simulink model "sldemo_variant_subsystems_enum"  (Simulink 7.6)
settings: Solver=FixedStepDiscrete  StartTime=0.0  StopTime=10.0  RelTol=1e-3
PreLoadFcn:
  | VSSE_NONLINEAR_CONTROLLER=Simulink.Variant('VSSE_MODE==sldemo_vss_CONTROLLER_TYPE.NONLINEAR')
  | VSSE_SECOND_ORDER_CONTROLLER=Simulink.Variant('VSSE_MODE==sldemo_vss_CONTROLLER_TYPE.SECOND_ORDER')
  | 
  | VSSE_MODE=sldemo_vss_CONTROLLER_TYPE.SECOND_ORDER
  | 
  | VSSE_PROTOTYPE = Simulink.Variant('VSSE_CURRENT_BUILD==sldemo_vss_BUILD_TYPE.PROTOTYPE')
  | VSSE_PRODUCTION = Simulink.Variant('VSSE_CURRENT_BUILD==sldemo_vss_BUILD_TYPE.PRODUCTION')
  | 
  | VSSE_CURRENT_BUILD=sldemo_vss_BUILD_TYPE.PRODUCTION
Description:
  | Variant Subsystems - Enumerations and Reuse
  | 
  | This demo illustrates Simulink(R) variant subsystems using enumerations
  | with Simulink.Variant objects. Variant subsystems let you provide multiple
  | implementations to a subsystem where only one implementation is active
  | during simulation. You can programmatically swap out the active
  | implementation and replace it with one of the other implementations
  | without modifying the model.
settings Model: Creator=The MathWorks Inc.
settings DataIOCC: SaveFormat=StructureWithTime
settings OptimizationCC: InlineParams=on
settings RTWCC: ProcessScript=grt_make_rtw_hook
settings CodeAppCC: MaxIdLength=100

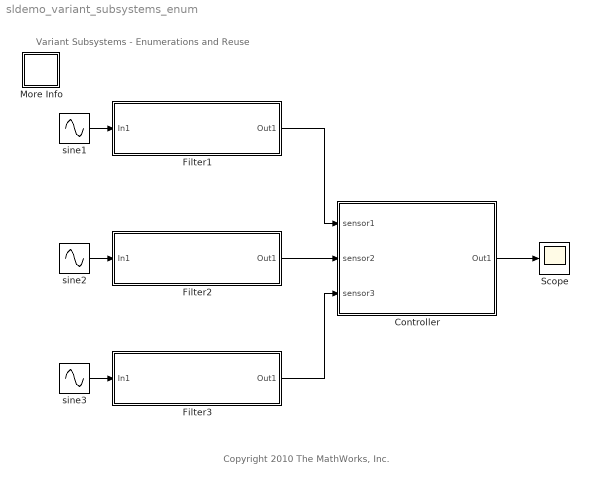
== system sldemo_variant_subsystems_enum ==
  note: Copyright 2010 The MathWorks, Inc.
  note: Variant Subsystems - Enumerations and Reuse
  Controller : Subsystem  Variant=on
  Filter1 : Subsystem  Variant=on
  Filter2 : Subsystem  Variant=on
  Filter3 : Subsystem  Variant=on
  More Info : Subsystem
      settings: OpenFcn=showdemo('sldemo_mdlref_variants')
      mask Display: disp('?')
  Scope : Scope
  sine1 : Sin  Amplitude=.1  Frequency=pi/3  SampleTime=.01
  sine2 : Sin  Amplitude=2  SampleTime=.01
  sine3 : Sin  Amplitude=.3  Frequency=pi/6  SampleTime=.01
  wires:
  sine2/1 -> Filter2/1(In1)
  sine1/1 -> Filter1/1(In1)
  sine3/1 -> Filter3/1(In1)
  Controller/1(Out1) -> Scope/1
  Filter3/1(Out1) -> Controller/3(sensor3)
  Filter2/1(Out1) -> Controller/2(sensor2)
  Filter1/1(Out1) -> Controller/1(sensor1)

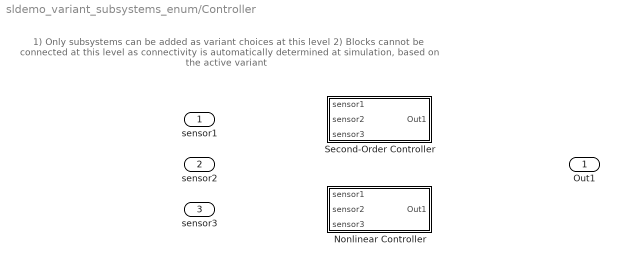
== system sldemo_variant_subsystems_enum/Controller ==
  note: 1) Only subsystems can be added as variant choices at this level
      | 2) Blocks cannot be connected at this level as connectivity is
      | automatically determined at simulation, based on the active variant
  sensor1 : Inport
  sensor2 : Inport  Port=2
  sensor3 : Inport  Port=3
  Nonlinear Controller : Subsystem  VariantObject=VSSE_NONLINEAR_CONTROLLER
  Second-Order Controller : Subsystem  VariantObject=VSSE_SECOND_ORDER_CONTROLLER
  Out1 : Outport

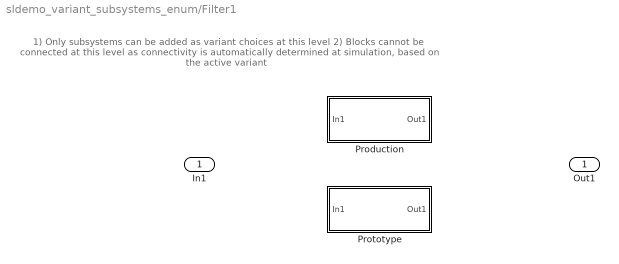
== system sldemo_variant_subsystems_enum/Filter1 ==
  note: 1) Only subsystems can be added as variant choices at this level
      | 2) Blocks cannot be connected at this level as connectivity is
      | automatically determined at simulation, based on the active variant
  In1 : Inport
  Production : Subsystem  VariantObject=VSSE_PRODUCTION
  Prototype : Subsystem  VariantObject=VSSE_PROTOTYPE
  Out1 : Outport

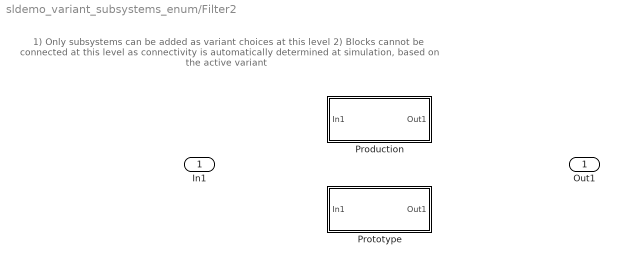
== system sldemo_variant_subsystems_enum/Filter2 ==
  note: 1) Only subsystems can be added as variant choices at this level
      | 2) Blocks cannot be connected at this level as connectivity is
      | automatically determined at simulation, based on the active variant
  In1 : Inport
  Production : Subsystem  VariantObject=VSSE_PRODUCTION
  Prototype : Subsystem  VariantObject=VSSE_PROTOTYPE
  Out1 : Outport

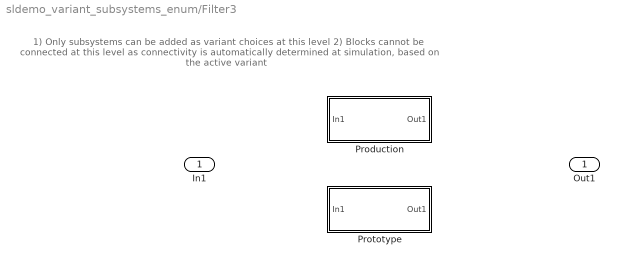
== system sldemo_variant_subsystems_enum/Filter3 ==
  note: 1) Only subsystems can be added as variant choices at this level
      | 2) Blocks cannot be connected at this level as connectivity is
      | automatically determined at simulation, based on the active variant
  In1 : Inport
  Production : Subsystem  VariantObject=VSSE_PRODUCTION
  Prototype : Subsystem  VariantObject=VSSE_PROTOTYPE
  Out1 : Outport

== system sldemo_variant_subsystems_enum/More Info ==
  note: Model Reference Variants - Enumerations and Reuse
  note: The following demo illustrates some Simulink.Variant capabilities
      |
      |    1. Enumerations: MATLAB enumeration classes can be used to improve
      |       readability in the conditions of the variant object.
      |
      |    2. Reuse: Simulink.Variant's can be reused in different Model blocks.

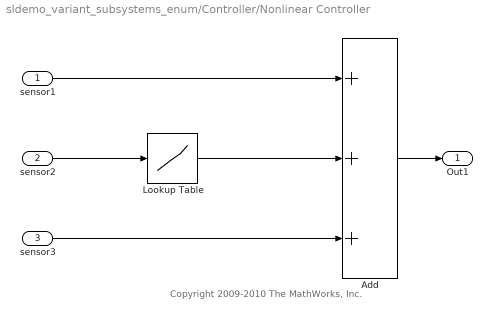
== system sldemo_variant_subsystems_enum/Controller/Nonlinear Controller ==
  note: Copyright 2009-2010 The MathWorks, Inc.
  sensor1 : Inport
  sensor2 : Inport  Port=2
  sensor3 : Inport  Port=3
  Add : Sum  Inputs=+++  SampleTime=.01
  Lookup Table : Lookup  InputValues=[-5:5]  Table=tanh([-5:5])
  Out1 : Outport
  wires:
  Add/1 -> Out1/1
  sensor1/1 -> Add/1
  sensor3/1 -> Add/3
  Lookup Table/1 -> Add/2
  sensor2/1 -> Lookup Table/1

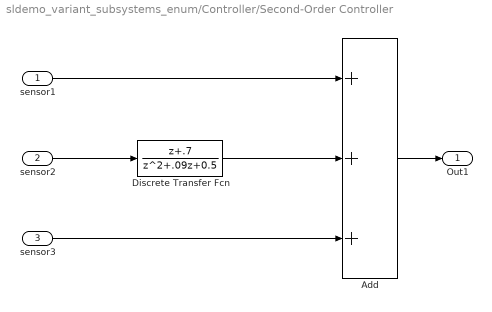
== system sldemo_variant_subsystems_enum/Controller/Second-Order Controller ==
  sensor1 : Inport
  sensor2 : Inport  Port=2
  sensor3 : Inport  Port=3
  Add : Sum  Inputs=+++
  Discrete Transfer Fcn : DiscreteTransferFcn  Numerator=[1 .7]  Denominator=[1 .09 0.5]  SampleTime=.01
  Out1 : Outport
  wires:
  Add/1 -> Out1/1
  sensor1/1 -> Add/1
  sensor3/1 -> Add/3
  Discrete Transfer Fcn/1 -> Add/2
  sensor2/1 -> Discrete Transfer Fcn/1

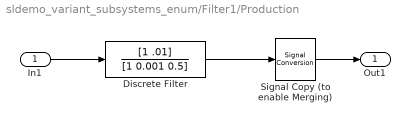
== system sldemo_variant_subsystems_enum/Filter1/Production ==
  In1 : Inport
  Discrete Filter : DiscreteFilter  Numerator=[1 .01]  Denominator=[1 0.001 0.5]  SampleTime=.01
  Signal Copy (to enable Merging) : SignalConversion  ConversionOutput=Contiguous copy
  Out1 : Outport
  wires:
  In1/1 -> Discrete Filter/1
  Discrete Filter/1 -> Signal Copy (to enable Merging)/1
  Signal Copy (to enable Merging)/1 -> Out1/1

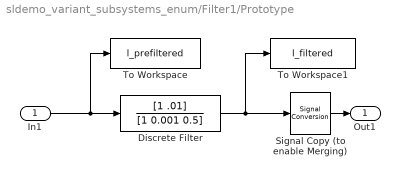
== system sldemo_variant_subsystems_enum/Filter1/Prototype ==
  In1 : Inport
  Discrete Filter : DiscreteFilter  Numerator=[1 .01]  Denominator=[1 0.001 0.5]  SampleTime=.01
  Signal Copy (to enable Merging) : SignalConversion  ConversionOutput=Contiguous copy
  To Workspace : ToWorkspace  VariableName=l_prefiltered  SampleTime=-1  SaveFormat=Structure
  To Workspace1 : ToWorkspace  VariableName=l_filtered  SampleTime=-1  SaveFormat=Structure
  Out1 : Outport
  wires:
  In1/1 -> To Workspace/1, Discrete Filter/1
  Discrete Filter/1 -> Signal Copy (to enable Merging)/1, To Workspace1/1
  Signal Copy (to enable Merging)/1 -> Out1/1

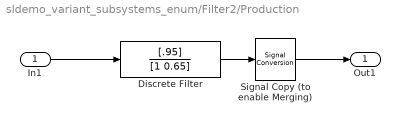
== system sldemo_variant_subsystems_enum/Filter2/Production ==
  In1 : Inport
  Discrete Filter : DiscreteFilter  Numerator=[.95]  Denominator=[1 0.65]  SampleTime=.01
  Signal Copy (to enable Merging) : SignalConversion  ConversionOutput=Contiguous copy
  Out1 : Outport
  wires:
  In1/1 -> Discrete Filter/1
  Discrete Filter/1 -> Signal Copy (to enable Merging)/1
  Signal Copy (to enable Merging)/1 -> Out1/1

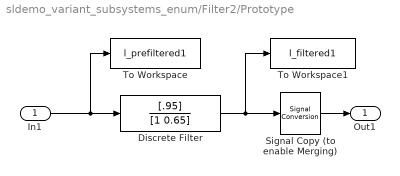
== system sldemo_variant_subsystems_enum/Filter2/Prototype ==
  In1 : Inport
  Discrete Filter : DiscreteFilter  Numerator=[.95]  Denominator=[1 0.65]  SampleTime=.01
  Signal Copy (to enable Merging) : SignalConversion  ConversionOutput=Contiguous copy
  To Workspace : ToWorkspace  VariableName=l_prefiltered1  SampleTime=-1  SaveFormat=Structure
  To Workspace1 : ToWorkspace  VariableName=l_filtered1  SampleTime=-1  SaveFormat=Structure
  Out1 : Outport
  wires:
  In1/1 -> To Workspace/1, Discrete Filter/1
  Discrete Filter/1 -> Signal Copy (to enable Merging)/1, To Workspace1/1
  Signal Copy (to enable Merging)/1 -> Out1/1

== system sldemo_variant_subsystems_enum/Filter3/Production ==
  In1 : Inport
  Discrete Filter : DiscreteFilter  SampleTime=.01
  Signal Copy (to enable Merging) : SignalConversion  ConversionOutput=Contiguous copy
  Out1 : Outport
  wires:
  In1/1 -> Discrete Filter/1
  Discrete Filter/1 -> Signal Copy (to enable Merging)/1
  Signal Copy (to enable Merging)/1 -> Out1/1

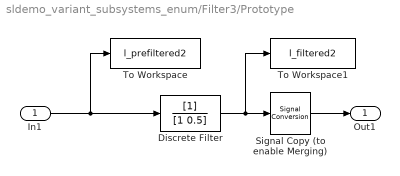
== system sldemo_variant_subsystems_enum/Filter3/Prototype ==
  In1 : Inport
  Discrete Filter : DiscreteFilter  SampleTime=.01
  Signal Copy (to enable Merging) : SignalConversion  ConversionOutput=Contiguous copy
  To Workspace : ToWorkspace  VariableName=l_prefiltered2  SampleTime=-1  SaveFormat=Structure
  To Workspace1 : ToWorkspace  VariableName=l_filtered2  SampleTime=-1  SaveFormat=Structure
  Out1 : Outport
  wires:
  In1/1 -> To Workspace/1, Discrete Filter/1
  Discrete Filter/1 -> Signal Copy (to enable Merging)/1, To Workspace1/1
  Signal Copy (to enable Merging)/1 -> Out1/1
